simulink model "TP_Bloc_Calcul_distribR2015a"  (R2015a)
settings: Solver=ode45  StartTime=0.0  StopTime=10.0  RelTol=1e-3
settings Model: CovModelRefEnable=off  Creator=eduardomendes  LastModifiedBy=eduardomendes
settings DataIOCC: LimitDataPoints=off  SaveFormat=Dataset
settings HardwareCC: ProdBitPerPointer=64  ProdLargestAtomicFloat=Float  ProdIntDivRoundTo=Zero  ProdEndianess=LittleEndian  ProdHWDeviceType=Specified
settings ModelReferenceCC: PropagateSignalLabelsOutOfModel=on

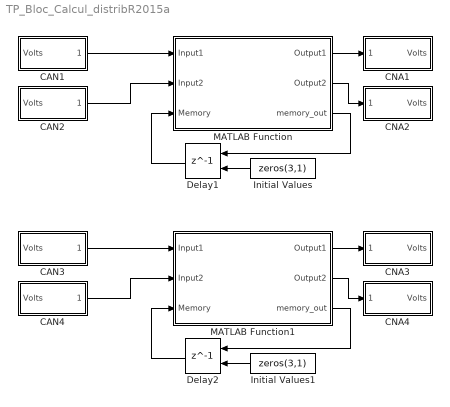
== system TP_Bloc_Calcul_distribR2015a ==
  CAN1 : Subsystem
  CAN2 : Subsystem
  CAN3 : Subsystem
  CAN4 : Subsystem
  CNA1 : Subsystem
  CNA2 : Subsystem
  CNA3 : Subsystem
  CNA4 : Subsystem
  Delay1 : Delay  DelayLength=1  InitialConditionSource=Input port  SampleTime=0.1
      settings: InputPortMap=u0,p4
  Delay2 : Delay  DelayLength=1  InitialConditionSource=Input port  SampleTime=0.1
      settings: InputPortMap=u0,p4
  Initial Values : Constant  Value=zeros(3,1)
  Initial Values1 : Constant  Value=zeros(3,1)
  MATLAB Function : MATLAB Function  TreatAsAtomicUnit=on  SystemSampleTime=0.01
      settings: PermitHierarchicalResolution=ParametersOnly
  MATLAB Function1 : MATLAB Function  TreatAsAtomicUnit=on  SystemSampleTime=0.01
      settings: PermitHierarchicalResolution=ParametersOnly
  wires:
  MATLAB Function/3(memory_out) -> Delay1/1
  Delay1/1 -> MATLAB Function/3(Memory)
  Initial Values/1 -> Delay1/2
  CAN2/1(N_8bits) -> MATLAB Function/2(Input2)
  CAN1/1(N_8bits) -> MATLAB Function/1(Input1)
  MATLAB Function/1(Output1) -> CNA1/1(N_8bits)
  MATLAB Function/2(Output2) -> CNA2/1(N_8bits)
  MATLAB Function1/3(memory_out) -> Delay2/1
  Delay2/1 -> MATLAB Function1/3(Memory)
  Initial Values1/1 -> Delay2/2
  CAN4/1(N_8bits) -> MATLAB Function1/2(Input2)
  CAN3/1(N_8bits) -> MATLAB Function1/1(Input1)
  MATLAB Function1/1(Output1) -> CNA3/1(N_8bits)
  MATLAB Function1/2(Output2) -> CNA4/1(N_8bits)

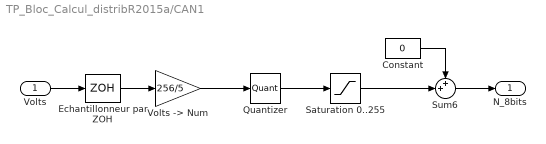
== system TP_Bloc_Calcul_distribR2015a/CAN1 ==
  Volts : Inport
  Constant : Constant  Value=0
  Echantillonneur par ZOH : ZeroOrderHold  SampleTime=0.1
  Quantizer : Quantizer  QuantizationInterval=1
  Saturation 0..255 : Saturate  UpperLimit=255  LowerLimit=0
  Sum6 : Sum  Inputs=++|  SaturateOnIntegerOverflow=on
  "Volts -> Num" : Gain  Gain=256/5  SaturateOnIntegerOverflow=on  OutDataTypeStr=Inherit: Same as input  ParamDataTypeStr=Inherit: Same as input
  N_8bits : Outport
  wires:
  Sum6/1 -> N_8bits/1
  Constant/1 -> Sum6/1
  Volts/1 -> Echantillonneur par ZOH/1
  "Volts -> Num"/1 -> Quantizer/1
  Saturation 0..255/1 -> Sum6/2
  Echantillonneur par ZOH/1 -> "Volts -> Num"/1
  Quantizer/1 -> Saturation 0..255/1

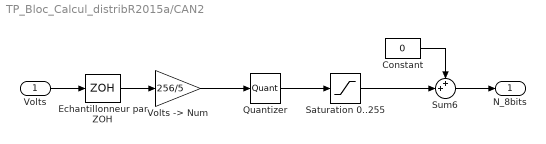
== system TP_Bloc_Calcul_distribR2015a/CAN2 ==
  Volts : Inport
  Constant : Constant  Value=0
  Echantillonneur par ZOH : ZeroOrderHold  SampleTime=0.1
  Quantizer : Quantizer  QuantizationInterval=1
  Saturation 0..255 : Saturate  UpperLimit=255  LowerLimit=0
  Sum6 : Sum  Inputs=++|  SaturateOnIntegerOverflow=on
  "Volts -> Num" : Gain  Gain=256/5  SaturateOnIntegerOverflow=on  OutDataTypeStr=Inherit: Same as input  ParamDataTypeStr=Inherit: Same as input
  N_8bits : Outport
  wires:
  Sum6/1 -> N_8bits/1
  Constant/1 -> Sum6/1
  Volts/1 -> Echantillonneur par ZOH/1
  "Volts -> Num"/1 -> Quantizer/1
  Saturation 0..255/1 -> Sum6/2
  Echantillonneur par ZOH/1 -> "Volts -> Num"/1
  Quantizer/1 -> Saturation 0..255/1

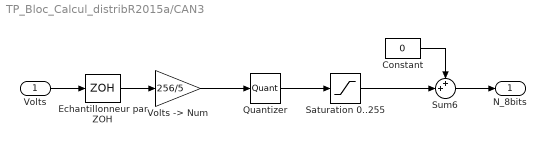
== system TP_Bloc_Calcul_distribR2015a/CAN3 ==
  Volts : Inport
  Constant : Constant  Value=0
  Echantillonneur par ZOH : ZeroOrderHold  SampleTime=0.1
  Quantizer : Quantizer  QuantizationInterval=1
  Saturation 0..255 : Saturate  UpperLimit=255  LowerLimit=0
  Sum6 : Sum  Inputs=++|  SaturateOnIntegerOverflow=on
  "Volts -> Num" : Gain  Gain=256/5  SaturateOnIntegerOverflow=on  OutDataTypeStr=Inherit: Same as input  ParamDataTypeStr=Inherit: Same as input
  N_8bits : Outport
  wires:
  Sum6/1 -> N_8bits/1
  Constant/1 -> Sum6/1
  Volts/1 -> Echantillonneur par ZOH/1
  "Volts -> Num"/1 -> Quantizer/1
  Saturation 0..255/1 -> Sum6/2
  Echantillonneur par ZOH/1 -> "Volts -> Num"/1
  Quantizer/1 -> Saturation 0..255/1

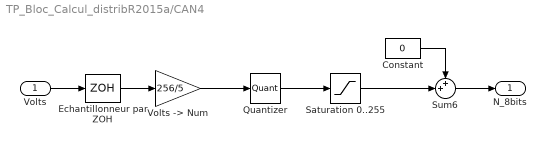
== system TP_Bloc_Calcul_distribR2015a/CAN4 ==
  Volts : Inport
  Constant : Constant  Value=0
  Echantillonneur par ZOH : ZeroOrderHold  SampleTime=0.1
  Quantizer : Quantizer  QuantizationInterval=1
  Saturation 0..255 : Saturate  UpperLimit=255  LowerLimit=0
  Sum6 : Sum  Inputs=++|  SaturateOnIntegerOverflow=on
  "Volts -> Num" : Gain  Gain=256/5  SaturateOnIntegerOverflow=on  OutDataTypeStr=Inherit: Same as input  ParamDataTypeStr=Inherit: Same as input
  N_8bits : Outport
  wires:
  Sum6/1 -> N_8bits/1
  Constant/1 -> Sum6/1
  Volts/1 -> Echantillonneur par ZOH/1
  "Volts -> Num"/1 -> Quantizer/1
  Saturation 0..255/1 -> Sum6/2
  Echantillonneur par ZOH/1 -> "Volts -> Num"/1
  Quantizer/1 -> Saturation 0..255/1

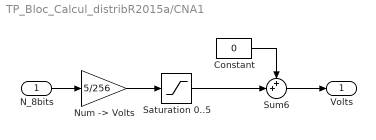
== system TP_Bloc_Calcul_distribR2015a/CNA1 ==
  N_8bits : Inport
  Constant : Constant  Value=0
  "Num -> Volts" : Gain  Gain=5/256  SaturateOnIntegerOverflow=on  OutDataTypeStr=Inherit: Same as input  ParamDataTypeStr=Inherit: Same as input
  Saturation 0..5 : Saturate  UpperLimit=5  LowerLimit=0
  Sum6 : Sum  Inputs=++|  SaturateOnIntegerOverflow=on
  Volts : Outport
  wires:
  Sum6/1 -> Volts/1
  Constant/1 -> Sum6/1
  N_8bits/1 -> "Num -> Volts"/1
  "Num -> Volts"/1 -> Saturation 0..5/1
  Saturation 0..5/1 -> Sum6/2

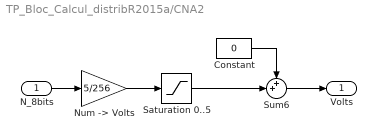
== system TP_Bloc_Calcul_distribR2015a/CNA2 ==
  N_8bits : Inport
  Constant : Constant  Value=0
  "Num -> Volts" : Gain  Gain=5/256  SaturateOnIntegerOverflow=on  OutDataTypeStr=Inherit: Same as input  ParamDataTypeStr=Inherit: Same as input
  Saturation 0..5 : Saturate  UpperLimit=5  LowerLimit=0
  Sum6 : Sum  Inputs=++|  SaturateOnIntegerOverflow=on
  Volts : Outport
  wires:
  Saturation 0..5/1 -> Sum6/2
  "Num -> Volts"/1 -> Saturation 0..5/1
  N_8bits/1 -> "Num -> Volts"/1
  Constant/1 -> Sum6/1
  Sum6/1 -> Volts/1

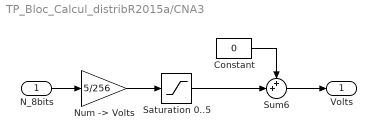
== system TP_Bloc_Calcul_distribR2015a/CNA3 ==
  N_8bits : Inport
  Constant : Constant  Value=0
  "Num -> Volts" : Gain  Gain=5/256  SaturateOnIntegerOverflow=on  OutDataTypeStr=Inherit: Same as input  ParamDataTypeStr=Inherit: Same as input
  Saturation 0..5 : Saturate  UpperLimit=5  LowerLimit=0
  Sum6 : Sum  Inputs=++|  SaturateOnIntegerOverflow=on
  Volts : Outport
  wires:
  Sum6/1 -> Volts/1
  Constant/1 -> Sum6/1
  N_8bits/1 -> "Num -> Volts"/1
  "Num -> Volts"/1 -> Saturation 0..5/1
  Saturation 0..5/1 -> Sum6/2

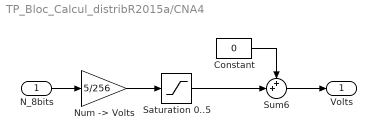
== system TP_Bloc_Calcul_distribR2015a/CNA4 ==
  N_8bits : Inport
  Constant : Constant  Value=0
  "Num -> Volts" : Gain  Gain=5/256  SaturateOnIntegerOverflow=on  OutDataTypeStr=Inherit: Same as input  ParamDataTypeStr=Inherit: Same as input
  Saturation 0..5 : Saturate  UpperLimit=5  LowerLimit=0
  Sum6 : Sum  Inputs=++|  SaturateOnIntegerOverflow=on
  Volts : Outport
  wires:
  Saturation 0..5/1 -> Sum6/2
  "Num -> Volts"/1 -> Saturation 0..5/1
  N_8bits/1 -> "Num -> Volts"/1
  Constant/1 -> Sum6/1
  Sum6/1 -> Volts/1

== matlab function TP_Bloc_Calcul_distribR2015a/MATLAB Function1 ==
  data: Input1 input; Input2 input; Output1 output; Output2 output; Memory input; memory_out output
function [Output1,Output2,memory_out] = Corr_Entier32(Input1,Input2,Memory)
% #codegen
%% File description
% Inputs : 
%   Input1 : consigne
%   Input2 : mesure
%   memory_in  : array of memorised values
%
% Outputs :
%   Output1 : commande
%   Output2 : consigne filtree
%	memory_out : array of values to be memorised

%% Parameters and variables
size_memory = 3;
memory_out = zeros(size_memory,1);

%% Processing

Q12 = 2^12;

% Read saved values
memory_in = Memory;
err_nm1   = memory_in(1);
y_nm1     = memory_in(2);
cons_fil_nm1   = memory_in(3);

% Passage de N 8bits Q8.0 à Q20.12
Input1Q12 = int32( Input1 * Q12);
Input2Q12 = int32( Input2 * Q12);

% Filtre de la consigne
cons_fil = Input1Q12 ;

% Correcteur
err = cons_fil - Input2Q12 ;
y  = err ;

% Saturation à Umax=5, Umin=0
if(y > int32(255*Q12)), y = int32(255*Q12); end;
if(y < int32(0*Q12)),   y = int32(0*Q12); end;

%% Outputs

% Sorties format Q8.0
Output1 = double(y/Q12) ;
Output2 = double(cons_fil/Q12) ; 

% Mémoires
memory_out(1) = err ;       % Save for next step
memory_out(2) = y ;         % Save for next step
memory_out(3) = cons_fil ;  % Save for next step

== matlab function TP_Bloc_Calcul_distribR2015a/MATLAB Function ==
  data: Input1 input; Input2 input; Output1 output; Output2 output; Memory input; memory_out output
function [Output1,Output2,memory_out] = Corr_float(Input1,Input2,Memory)
% #codegen
%% File description
% Inputs : 
%   Input1 : consigne
%   Input2 : mesure
%   memory_in  : array of memorised values
%
% Outputs :
%   Output1 : commande
%   Output2 : consigne filtree
%	memory_out : array of values to be memorised

%% Parameters and variables
size_memory = 3;
memory_out = zeros(size_memory,1);

%% Processing

% Read saved values
memory_in = Memory;
err_nm1   = memory_in(1);
y_nm1     = memory_in(2);
cons_fil_nm1 = memory_in(3);


% Passage de N 8bits Q8.0 à 0..5volts
Input1 = 5/256*Input1;
Input2 = 5/256*Input2;

% Filtre de la consigne
cons_fil = Input1 ;

% Correcteur 
err = cons_fil - Input2 ;
y  = err ;

% Saturation à Umax=5, Umin=0
if(y > 5), y = 5; end;
if(y < 0), y = 0; end;

%% Outputs

% Sorties format Q8.0
Output1 = round(255/5*y) ;
Output2 = round(255/5*cons_fil) ; 

% Mémoires
memory_out(1) = err ;       % Save for next step
memory_out(2) = y ;         % Save for next step
memory_out(3) = cons_fil ;  % Save for next step
